simulink model "DriveSystemControl"  (R2023b)
settings: Solver=FixedStepAuto  StartTime=0.0  StopTime=Inf  FixedStep=0.001  RelTol=1e-3
PostLoadFcn:
  | if any(exist('dsrtsu_mdlpostloadfcn', 'file') ~= 0), dsrtsu_mdlpostloadfcn('Execute', bdroot); end
InitFcn:
  | , if any(exist('rtifpga_mdlclblib', 'file') ~= 0), rtifpga_mdlclblib('Init', bdroot); end,
  | , if any(exist('dsmpb_private', 'file') ~= 0), dsmpb_private('dsmpb_mdlclblib', 'Init', bdroot); end,
libraries: dsmpblib x2
(part 6 of 11)

== system DriveSystemControl/Bus Configuration (1) - Out/Simulated ECUs/Virya Controller CAN File 08082024/Telematics/RX/PDUs/TCU03/sigCurrentSensorFault ==
  sigCurrentSensorFault : Inport
  ISignal Value : Subsystem
  _sigCurrentSensorFault_ : BusSelector  OutputSignals=ISignal Value
  wires:
  sigCurrentSensorFault/1 -> _sigCurrentSensorFault_/1  "sigCurrentSensorFault"
  _sigCurrentSensorFault_/1 -> ISignal Value/1(ISignal Value)  "<ISignal Value>"

== system DriveSystemControl/Bus Configuration (1) - Out/Simulated ECUs/Virya Controller CAN File 08082024/Telematics/RX/PDUs/TCU03/sigEEPROMFailure ==
  sigEEPROMFailure : Inport
  ISignal Value : Subsystem
  _sigEEPROMFailure_ : BusSelector  OutputSignals=ISignal Value
  wires:
  sigEEPROMFailure/1 -> _sigEEPROMFailure_/1  "sigEEPROMFailure"
  _sigEEPROMFailure_/1 -> ISignal Value/1(ISignal Value)  "<ISignal Value>"

== system DriveSystemControl/Bus Configuration (1) - Out/Simulated ECUs/Virya Controller CAN File 08082024/Telematics/RX/PDUs/TCU03/sigHighPedalDisable ==
  sigHighPedalDisable : Inport
  ISignal Value : Subsystem
  _sigHighPedalDisable_ : BusSelector  OutputSignals=ISignal Value
  wires:
  sigHighPedalDisable/1 -> _sigHighPedalDisable_/1  "sigHighPedalDisable"
  _sigHighPedalDisable_/1 -> ISignal Value/1(ISignal Value)  "<ISignal Value>"

== system DriveSystemControl/Bus Configuration (1) - Out/Simulated ECUs/Virya Controller CAN File 08082024/Telematics/RX/PDUs/TCU03/sigInsulationResistanceLow ==
  sigInsulationResistanceLow : Inport
  ISignal Value : Subsystem
  _sigInsulationResistanceLow_ : BusSelector  OutputSignals=ISignal Value
  wires:
  sigInsulationResistanceLow/1 -> _sigInsulationResistanceLow_/1  "sigInsulationResistanceLow"
  _sigInsulationResistanceLow_/1 -> ISignal Value/1(ISignal Value)  "<ISignal Value>"

== system DriveSystemControl/Bus Configuration (1) - Out/Simulated ECUs/Virya Controller CAN File 08082024/Telematics/RX/PDUs/TCU03/sigMainContactorWelded ==
  sigMainContactorWelded : Inport
  ISignal Value : Subsystem
  _sigMainContactorWelded_ : BusSelector  OutputSignals=ISignal Value
  wires:
  sigMainContactorWelded/1 -> _sigMainContactorWelded_/1  "sigMainContactorWelded"
  _sigMainContactorWelded_/1 -> ISignal Value/1(ISignal Value)  "<ISignal Value>"

== system DriveSystemControl/Bus Configuration (1) - Out/Simulated ECUs/Virya Controller CAN File 08082024/Telematics/RX/PDUs/TCU03/sigMainContactordidnotClose ==
  sigMainContactordidnotClose : Inport
  ISignal Value : Subsystem
  _sigMainContactordidnotClose_ : BusSelector  OutputSignals=ISignal Value
  wires:
  sigMainContactordidnotClose/1 -> _sigMainContactordidnotClose_/1  "sigMainContactordidnotClose"
  _sigMainContactordidnotClose_/1 -> ISignal Value/1(ISignal Value)  "<ISignal Value>"

== system DriveSystemControl/Bus Configuration (1) - Out/Simulated ECUs/Virya Controller CAN File 08082024/Telematics/RX/PDUs/TCU03/sigMainOpenShort ==
  sigMainOpenShort : Inport
  ISignal Value : Subsystem
  _sigMainOpenShort_ : BusSelector  OutputSignals=ISignal Value
  wires:
  sigMainOpenShort/1 -> _sigMainOpenShort_/1  "sigMainOpenShort"
  _sigMainOpenShort_/1 -> ISignal Value/1(ISignal Value)  "<ISignal Value>"

== system DriveSystemControl/Bus Configuration (1) - Out/Simulated ECUs/Virya Controller CAN File 08082024/Telematics/RX/PDUs/TCU03/sigMotorCharacterization ==
  sigMotorCharacterization : Inport
  ISignal Value : Subsystem
  _sigMotorCharacterization_ : BusSelector  OutputSignals=ISignal Value
  wires:
  sigMotorCharacterization/1 -> _sigMotorCharacterization_/1  "sigMotorCharacterization"
  _sigMotorCharacterization_/1 -> ISignal Value/1(ISignal Value)  "<ISignal Value>"

== system DriveSystemControl/Bus Configuration (1) - Out/Simulated ECUs/Virya Controller CAN File 08082024/Telematics/RX/PDUs/TCU03/sigMotorPhaseOpen ==
  sigMotorPhaseOpen : Inport
  ISignal Value : Subsystem
  _sigMotorPhaseOpen_ : BusSelector  OutputSignals=ISignal Value
  wires:
  sigMotorPhaseOpen/1 -> _sigMotorPhaseOpen_/1  "sigMotorPhaseOpen"
  _sigMotorPhaseOpen_/1 -> ISignal Value/1(ISignal Value)  "<ISignal Value>"

== system DriveSystemControl/Bus Configuration (1) - Out/Simulated ECUs/Virya Controller CAN File 08082024/Telematics/RX/PDUs/TCU03/sigMotorTempHotCutback ==
  sigMotorTempHotCutback : Inport
  ISignal Value : Subsystem
  _sigMotorTempHotCutback_ : BusSelector  OutputSignals=ISignal Value
  wires:
  sigMotorTempHotCutback/1 -> _sigMotorTempHotCutback_/1  "sigMotorTempHotCutback"
  _sigMotorTempHotCutback_/1 -> ISignal Value/1(ISignal Value)  "<ISignal Value>"

== system DriveSystemControl/Bus Configuration (1) - Out/Simulated ECUs/Virya Controller CAN File 08082024/Telematics/RX/PDUs/TCU03/sigMotorTempSensorFault ==
  sigMotorTempSensorFault : Inport
  ISignal Value : Subsystem
  _sigMotorTempSensorFault_ : BusSelector  OutputSignals=ISignal Value
  wires:
  sigMotorTempSensorFault/1 -> _sigMotorTempSensorFault_/1  "sigMotorTempSensorFault"
  _sigMotorTempSensorFault_/1 -> ISignal Value/1(ISignal Value)  "<ISignal Value>"

== system DriveSystemControl/Bus Configuration (1) - Out/Simulated ECUs/Virya Controller CAN File 08082024/Telematics/RX/PDUs/TCU03/sigOEM_BatterySTOPSignal ==
  sigOEM_BatterySTOPSignal : Inport
  ISignal Value : Subsystem
  _sigOEM_BatterySTOPSignal_ : BusSelector  OutputSignals=ISignal Value
  wires:
  sigOEM_BatterySTOPSignal/1 -> _sigOEM_BatterySTOPSignal_/1  "sigOEM_BatterySTOPSignal"
  _sigOEM_BatterySTOPSignal_/1 -> ISignal Value/1(ISignal Value)  "<ISignal Value>"

== system DriveSystemControl/Bus Configuration (1) - Out/Simulated ECUs/Virya Controller CAN File 08082024/Telematics/RX/PDUs/TCU03/sigOEM_NoBatteryCAN ==
  sigOEM_NoBatteryCAN : Inport
  ISignal Value : Subsystem
  _sigOEM_NoBatteryCAN_ : BusSelector  OutputSignals=ISignal Value
  wires:
  sigOEM_NoBatteryCAN/1 -> _sigOEM_NoBatteryCAN_/1  "sigOEM_NoBatteryCAN"
  _sigOEM_NoBatteryCAN_/1 -> ISignal Value/1(ISignal Value)  "<ISignal Value>"

== system DriveSystemControl/Bus Configuration (1) - Out/Simulated ECUs/Virya Controller CAN File 08082024/Telematics/RX/PDUs/TCU03/sigOSGeneral ==
  sigOSGeneral : Inport
  ISignal Value : Subsystem
  _sigOSGeneral_ : BusSelector  OutputSignals=ISignal Value
  wires:
  sigOSGeneral/1 -> _sigOSGeneral_/1  "sigOSGeneral"
  _sigOSGeneral_/1 -> ISignal Value/1(ISignal Value)  "<ISignal Value>"

== system DriveSystemControl/Bus Configuration (1) - Out/Simulated ECUs/Virya Controller CAN File 08082024/Telematics/RX/PDUs/TCU03/sigPMACCommissioningNeeded ==
  sigPMACCommissioningNeeded : Inport
  ISignal Value : Subsystem
  _sigPMACCommissioningNeeded_ : BusSelector  OutputSignals=ISignal Value
  wires:
  sigPMACCommissioningNeeded/1 -> _sigPMACCommissioningNeeded_/1  "sigPMACCommissioningNeeded"
  _sigPMACCommissioningNeeded_/1 -> ISignal Value/1(ISignal Value)  "<ISignal Value>"

== system DriveSystemControl/Bus Configuration (1) - Out/Simulated ECUs/Virya Controller CAN File 08082024/Telematics/RX/PDUs/TCU03/sigParameterChangeFault ==
  sigParameterChangeFault : Inport
  ISignal Value : Subsystem
  _sigParameterChangeFault_ : BusSelector  OutputSignals=ISignal Value
  wires:
  sigParameterChangeFault/1 -> _sigParameterChangeFault_/1  "sigParameterChangeFault"
  _sigParameterChangeFault_/1 -> ISignal Value/1(ISignal Value)  "<ISignal Value>"

== system DriveSystemControl/Bus Configuration (1) - Out/Simulated ECUs/Virya Controller CAN File 08082024/Telematics/RX/PDUs/TCU03/sigPhasePWMMismatch ==
  sigPhasePWMMismatch : Inport
  ISignal Value : Subsystem
  _sigPhasePWMMismatch_ : BusSelector  OutputSignals=ISignal Value
  wires:
  sigPhasePWMMismatch/1 -> _sigPhasePWMMismatch_/1  "sigPhasePWMMismatch"
  _sigPhasePWMMismatch_/1 -> ISignal Value/1(ISignal Value)  "<ISignal Value>"

== system DriveSystemControl/Bus Configuration (1) - Out/Simulated ECUs/Virya Controller CAN File 08082024/Telematics/RX/PDUs/TCU03/sigPrechargeFailed ==
  sigPrechargeFailed : Inport
  ISignal Value : Subsystem
  _sigPrechargeFailed_ : BusSelector  OutputSignals=ISignal Value
  wires:
  sigPrechargeFailed/1 -> _sigPrechargeFailed_/1  "sigPrechargeFailed"
  _sigPrechargeFailed_/1 -> ISignal Value/1(ISignal Value)  "<ISignal Value>"

== system DriveSystemControl/Bus Configuration (1) - Out/Simulated ECUs/Virya Controller CAN File 08082024/Telematics/RX/PDUs/TCU03/sigSevereBPosOvervoltage ==
  sigSevereBPosOvervoltage : Inport
  ISignal Value : Subsystem
  _sigSevereBPosOvervoltage_ : BusSelector  OutputSignals=ISignal Value
  wires:
  sigSevereBPosOvervoltage/1 -> _sigSevereBPosOvervoltage_/1  "sigSevereBPosOvervoltage"
  _sigSevereBPosOvervoltage_/1 -> ISignal Value/1(ISignal Value)  "<ISignal Value>"

== system DriveSystemControl/Bus Configuration (1) - Out/Simulated ECUs/Virya Controller CAN File 08082024/Telematics/RX/PDUs/TCU03/sigSevereBPosUndervoltage ==
  sigSevereBPosUndervoltage : Inport
  ISignal Value : Subsystem
  _sigSevereBPosUndervoltage_ : BusSelector  OutputSignals=ISignal Value
  wires:
  sigSevereBPosUndervoltage/1 -> _sigSevereBPosUndervoltage_/1  "sigSevereBPosUndervoltage"
  _sigSevereBPosUndervoltage_/1 -> ISignal Value/1(ISignal Value)  "<ISignal Value>"

== system DriveSystemControl/Bus Configuration (1) - Out/Simulated ECUs/Virya Controller CAN File 08082024/Telematics/RX/PDUs/TCU03/sigSevereKSIOvervoltage ==
  sigSevereKSIOvervoltage : Inport
  ISignal Value : Subsystem
  _sigSevereKSIOvervoltage_ : BusSelector  OutputSignals=ISignal Value
  wires:
  sigSevereKSIOvervoltage/1 -> _sigSevereKSIOvervoltage_/1  "sigSevereKSIOvervoltage"
  _sigSevereKSIOvervoltage_/1 -> ISignal Value/1(ISignal Value)  "<ISignal Value>"

== system DriveSystemControl/Bus Configuration (1) - Out/Simulated ECUs/Virya Controller CAN File 08082024/Telematics/RX/PDUs/TCU03/sigSevereKSIUndervoltage ==
  sigSevereKSIUndervoltage : Inport
  ISignal Value : Subsystem
  _sigSevereKSIUndervoltage_ : BusSelector  OutputSignals=ISignal Value
  wires:
  sigSevereKSIUndervoltage/1 -> _sigSevereKSIUndervoltage_/1  "sigSevereKSIUndervoltage"
  _sigSevereKSIUndervoltage_/1 -> ISignal Value/1(ISignal Value)  "<ISignal Value>"

== system DriveSystemControl/Bus Configuration (1) - Out/Simulated ECUs/Virya Controller CAN File 08082024/Telematics/RX/PDUs/TCU03/sigSinCosMisalignment ==
  sigSinCosMisalignment : Inport
  ISignal Value : Subsystem
  _sigSinCosMisalignment_ : BusSelector  OutputSignals=ISignal Value
  wires:
  sigSinCosMisalignment/1 -> _sigSinCosMisalignment_/1  "sigSinCosMisalignment"
  _sigSinCosMisalignment_/1 -> ISignal Value/1(ISignal Value)  "<ISignal Value>"

== system DriveSystemControl/Bus Configuration (1) - Out/Simulated ECUs/Virya Controller CAN File 08082024/Telematics/RX/PDUs/TCU03/sigSinCosSensorFault ==
  sigSinCosSensorFault : Inport
  ISignal Value : Subsystem
  _sigSinCosSensorFault_ : BusSelector  OutputSignals=ISignal Value
  wires:
  sigSinCosSensorFault/1 -> _sigSinCosSensorFault_/1  "sigSinCosSensorFault"
  _sigSinCosSensorFault_/1 -> ISignal Value/1(ISignal Value)  "<ISignal Value>"

== system DriveSystemControl/Bus Configuration (1) - Out/Simulated ECUs/Virya Controller CAN File 08082024/Telematics/RX/PDUs/TCU03/sigStallDetected ==
  sigStallDetected : Inport
  ISignal Value : Subsystem
  _sigStallDetected_ : BusSelector  OutputSignals=ISignal Value
  wires:
  sigStallDetected/1 -> _sigStallDetected_/1  "sigStallDetected"
  _sigStallDetected_/1 -> ISignal Value/1(ISignal Value)  "<ISignal Value>"

== system DriveSystemControl/Bus Configuration (1) - Out/Simulated ECUs/Virya Controller CAN File 08082024/Telematics/RX/PDUs/TCU03/sigSupervisorFault ==
  sigSupervisorFault : Inport
  ISignal Value : Subsystem
  _sigSupervisorFault_ : BusSelector  OutputSignals=ISignal Value
  wires:
  sigSupervisorFault/1 -> _sigSupervisorFault_/1  "sigSupervisorFault"
  _sigSupervisorFault_/1 -> ISignal Value/1(ISignal Value)  "<ISignal Value>"

== system DriveSystemControl/Bus Configuration (1) - Out/Simulated ECUs/Virya Controller CAN File 08082024/Telematics/RX/PDUs/TCU03/sigThrottlewiperHigh ==
  sigThrottlewiperHigh : Inport
  ISignal Value : Subsystem
  _sigThrottlewiperHigh_ : BusSelector  OutputSignals=ISignal Value
  wires:
  sigThrottlewiperHigh/1 -> _sigThrottlewiperHigh_/1  "sigThrottlewiperHigh"
  _sigThrottlewiperHigh_/1 -> ISignal Value/1(ISignal Value)  "<ISignal Value>"

== system DriveSystemControl/Bus Configuration (1) - Out/Simulated ECUs/Virya Controller CAN File 08082024/Telematics/RX/PDUs/TCU03/sigThrottlewiperLow ==
  sigThrottlewiperLow : Inport
  ISignal Value : Subsystem
  _sigThrottlewiperLow_ : BusSelector  OutputSignals=ISignal Value
  wires:
  sigThrottlewiperLow/1 -> _sigThrottlewiperLow_/1  "sigThrottlewiperLow"
  _sigThrottlewiperLow_/1 -> ISignal Value/1(ISignal Value)  "<ISignal Value>"

== system DriveSystemControl/Bus Configuration (1) - Out/Simulated ECUs/Virya Controller CAN File 08082024/Telematics/RX/PDUs/TCU03/sigVCLRunTimeError ==
  sigVCLRunTimeError : Inport
  ISignal Value : Subsystem
  _sigVCLRunTimeError_ : BusSelector  OutputSignals=ISignal Value
  wires:
  sigVCLRunTimeError/1 -> _sigVCLRunTimeError_/1  "sigVCLRunTimeError"
  _sigVCLRunTimeError_/1 -> ISignal Value/1(ISignal Value)  "<ISignal Value>"

== system DriveSystemControl/Bus Configuration (1) - Out/Simulated ECUs/Virya Controller CAN File 08082024/Telematics/RX/PDUs/TCU04/sigMCU5_DriveMode ==
  sigMCU5_DriveMode : Inport
  ISignal Value : Subsystem
  _sigMCU5_DriveMode_ : BusSelector  OutputSignals=ISignal Value
  wires:
  sigMCU5_DriveMode/1 -> _sigMCU5_DriveMode_/1  "sigMCU5_DriveMode"
  _sigMCU5_DriveMode_/1 -> ISignal Value/1(ISignal Value)  "<ISignal Value>"

== system DriveSystemControl/Bus Configuration (1) - Out/Simulated ECUs/Virya Controller CAN File 08082024/Telematics/RX/PDUs/TCU04/sigMCU5_Efficiency ==
  sigMCU5_Efficiency : Inport
  ISignal Value : Subsystem
  _sigMCU5_Efficiency_ : BusSelector  OutputSignals=ISignal Value
  wires:
  sigMCU5_Efficiency/1 -> _sigMCU5_Efficiency_/1  "sigMCU5_Efficiency"
  _sigMCU5_Efficiency_/1 -> ISignal Value/1(ISignal Value)  "<ISignal Value>"

== system DriveSystemControl/Bus Configuration (1) - Out/Simulated ECUs/Virya Controller CAN File 08082024/Telematics/RX/PDUs/TCU04/sigMCU5_Hillhold ==
  sigMCU5_Hillhold : Inport
  ISignal Value : Subsystem
  _sigMCU5_Hillhold_ : BusSelector  OutputSignals=ISignal Value
  wires:
  sigMCU5_Hillhold/1 -> _sigMCU5_Hillhold_/1  "sigMCU5_Hillhold"
  _sigMCU5_Hillhold_/1 -> ISignal Value/1(ISignal Value)  "<ISignal Value>"

== system DriveSystemControl/Bus Configuration (1) - Out/Simulated ECUs/Virya Controller CAN File 08082024/Telematics/RX/PDUs/TCU04/sigMCU5_RegenFlag ==
  sigMCU5_RegenFlag : Inport
  ISignal Value : Subsystem
  _sigMCU5_RegenFlag_ : BusSelector  OutputSignals=ISignal Value
  wires:
  sigMCU5_RegenFlag/1 -> _sigMCU5_RegenFlag_/1  "sigMCU5_RegenFlag"
  _sigMCU5_RegenFlag_/1 -> ISignal Value/1(ISignal Value)  "<ISignal Value>"

== system DriveSystemControl/Bus Configuration (1) - Out/Simulated ECUs/Virya Controller CAN File 08082024/Telematics/RX/PDUs/TCU04/sigMCU5_Speed ==
  sigMCU5_Speed : Inport
  ISignal Value : Subsystem
  _sigMCU5_Speed_ : BusSelector  OutputSignals=ISignal Value
  wires:
  sigMCU5_Speed/1 -> _sigMCU5_Speed_/1  "sigMCU5_Speed"
  _sigMCU5_Speed_/1 -> ISignal Value/1(ISignal Value)  "<ISignal Value>"

== system DriveSystemControl/Bus Configuration (1) - Out/Simulated ECUs/Virya Controller CAN File 08082024/Telematics/RX/PDUs/TCU05/sigMCU6_Odometer ==
  sigMCU6_Odometer : Inport
  ISignal Value : Subsystem
  _sigMCU6_Odometer_ : BusSelector  OutputSignals=ISignal Value
  wires:
  sigMCU6_Odometer/1 -> _sigMCU6_Odometer_/1  "sigMCU6_Odometer"
  _sigMCU6_Odometer_/1 -> ISignal Value/1(ISignal Value)  "<ISignal Value>"

== system DriveSystemControl/Bus Configuration (1) - In/Manipulation/Virya Controller CAN File 08082024/WIP/CANChannel/PDUs/BMS01/sigBatteryMalfunctionLight/Feature Switch ==
  Const_sigBatteryMalfunctionLight Countdown Start Value : Constant  Value=0  OutDataTypeStr=uint32
  Const_sigBatteryMalfunctionLight Feature Switch : Constant  Value=0  OutDataTypeStr=uint32
  _Feature Switch_ : BusCreator  Inputs=2
  Feature Switch : Outport
  wires:
  _Feature Switch_/1 -> Feature Switch/1  "Feature Switch"
  Const_sigBatteryMalfunctionLight Countdown Start Value/1 -> _Feature Switch_/1  "sigBatteryMalfunctionLight Countdown Start Value"
  Const_sigBatteryMalfunctionLight Feature Switch/1 -> _Feature Switch_/2  "sigBatteryMalfunctionLight Feature Switch"

== system DriveSystemControl/Bus Configuration (1) - In/Manipulation/Virya Controller CAN File 08082024/WIP/CANChannel/PDUs/BMS01/sigBatteryMalfunctionLight/ISignal Overwrite Value ==
  Const_sigBatteryMalfunctionLight Overwrite Value : Constant  Value=0  OutDataTypeStr=uint8
  _ISignal Overwrite Value_ : BusCreator  Inputs=1
  ISignal Overwrite Value : Outport
  wires:
  _ISignal Overwrite Value_/1 -> ISignal Overwrite Value/1  "ISignal Overwrite Value"
  Const_sigBatteryMalfunctionLight Overwrite Value/1 -> _ISignal Overwrite Value_/1  "sigBatteryMalfunctionLight Overwrite Value"

== system DriveSystemControl/Bus Configuration (1) - In/Manipulation/Virya Controller CAN File 08082024/WIP/CANChannel/PDUs/BMS01/sigKeyOnIndicator/Feature Switch ==
  Const_sigKeyOnIndicator Countdown Start Value : Constant  Value=0  OutDataTypeStr=uint32
  Const_sigKeyOnIndicator Feature Switch : Constant  Value=0  OutDataTypeStr=uint32
  _Feature Switch_ : BusCreator  Inputs=2
  Feature Switch : Outport
  wires:
  _Feature Switch_/1 -> Feature Switch/1  "Feature Switch"
  Const_sigKeyOnIndicator Countdown Start Value/1 -> _Feature Switch_/1  "sigKeyOnIndicator Countdown Start Value"
  Const_sigKeyOnIndicator Feature Switch/1 -> _Feature Switch_/2  "sigKeyOnIndicator Feature Switch"

== system DriveSystemControl/Bus Configuration (1) - In/Manipulation/Virya Controller CAN File 08082024/WIP/CANChannel/PDUs/BMS01/sigKeyOnIndicator/ISignal Overwrite Value ==
  Const_sigKeyOnIndicator Overwrite Value : Constant  Value=0  OutDataTypeStr=uint8
  _ISignal Overwrite Value_ : BusCreator  Inputs=1
  ISignal Overwrite Value : Outport
  wires:
  _ISignal Overwrite Value_/1 -> ISignal Overwrite Value/1  "ISignal Overwrite Value"
  Const_sigKeyOnIndicator Overwrite Value/1 -> _ISignal Overwrite Value_/1  "sigKeyOnIndicator Overwrite Value"

== system DriveSystemControl/Bus Configuration (1) - In/Manipulation/Virya Controller CAN File 08082024/WIP/CANChannel/PDUs/BMS01/sigStateOfCharge/Feature Switch ==
  Const_sigStateOfCharge Countdown Start Value : Constant  Value=0  OutDataTypeStr=uint32
  Const_sigStateOfCharge Feature Switch : Constant  Value=0  OutDataTypeStr=uint32
  _Feature Switch_ : BusCreator  Inputs=2
  Feature Switch : Outport
  wires:
  _Feature Switch_/1 -> Feature Switch/1  "Feature Switch"
  Const_sigStateOfCharge Countdown Start Value/1 -> _Feature Switch_/1  "sigStateOfCharge Countdown Start Value"
  Const_sigStateOfCharge Feature Switch/1 -> _Feature Switch_/2  "sigStateOfCharge Feature Switch"

== system DriveSystemControl/Bus Configuration (1) - In/Manipulation/Virya Controller CAN File 08082024/WIP/CANChannel/PDUs/BMS01/sigStateOfCharge/ISignal Overwrite Value ==
  Const_sigStateOfCharge Overwrite Value : Constant  Value=0  OutDataTypeStr=uint8
  _ISignal Overwrite Value_ : BusCreator  Inputs=1
  ISignal Overwrite Value : Outport
  wires:
  _ISignal Overwrite Value_/1 -> ISignal Overwrite Value/1  "ISignal Overwrite Value"
  Const_sigStateOfCharge Overwrite Value/1 -> _ISignal Overwrite Value_/1  "sigStateOfCharge Overwrite Value"

== system DriveSystemControl/Bus Configuration (1) - In/Manipulation/Virya Controller CAN File 08082024/WIP/CANChannel/PDUs/BMS02/sigBatteryCurrent/Feature Switch ==
  Const_sigBatteryCurrent Countdown Start Value : Constant  Value=0  OutDataTypeStr=uint32
  Const_sigBatteryCurrent Feature Switch : Constant  Value=0  OutDataTypeStr=uint32
  _Feature Switch_ : BusCreator  Inputs=2
  Feature Switch : Outport
  wires:
  _Feature Switch_/1 -> Feature Switch/1  "Feature Switch"
  Const_sigBatteryCurrent Countdown Start Value/1 -> _Feature Switch_/1  "sigBatteryCurrent Countdown Start Value"
  Const_sigBatteryCurrent Feature Switch/1 -> _Feature Switch_/2  "sigBatteryCurrent Feature Switch"

== system DriveSystemControl/Bus Configuration (1) - In/Manipulation/Virya Controller CAN File 08082024/WIP/CANChannel/PDUs/BMS02/sigBatteryCurrent/ISignal Overwrite Value ==
  Const_sigBatteryCurrent Overwrite Value : Constant  Value=0  OutDataTypeStr=double
  _ISignal Overwrite Value_ : BusCreator  Inputs=1
  ISignal Overwrite Value : Outport
  wires:
  _ISignal Overwrite Value_/1 -> ISignal Overwrite Value/1  "ISignal Overwrite Value"
  Const_sigBatteryCurrent Overwrite Value/1 -> _ISignal Overwrite Value_/1  "sigBatteryCurrent Overwrite Value"

== system DriveSystemControl/Bus Configuration (1) - In/Manipulation/Virya Controller CAN File 08082024/WIP/CANChannel/PDUs/BMS02/sigDriveCurrentLimit/Feature Switch ==
  Const_sigDriveCurrentLimit Countdown Start Value : Constant  Value=0  OutDataTypeStr=uint32
  Const_sigDriveCurrentLimit Feature Switch : Constant  Value=0  OutDataTypeStr=uint32
  _Feature Switch_ : BusCreator  Inputs=2
  Feature Switch : Outport
  wires:
  _Feature Switch_/1 -> Feature Switch/1  "Feature Switch"
  Const_sigDriveCurrentLimit Countdown Start Value/1 -> _Feature Switch_/1  "sigDriveCurrentLimit Countdown Start Value"
  Const_sigDriveCurrentLimit Feature Switch/1 -> _Feature Switch_/2  "sigDriveCurrentLimit Feature Switch"

== system DriveSystemControl/Bus Configuration (1) - In/Manipulation/Virya Controller CAN File 08082024/WIP/CANChannel/PDUs/BMS02/sigDriveCurrentLimit/ISignal Overwrite Value ==
  Const_sigDriveCurrentLimit Overwrite Value : Constant  Value=0  OutDataTypeStr=uint8
  _ISignal Overwrite Value_ : BusCreator  Inputs=1
  ISignal Overwrite Value : Outport
  wires:
  _ISignal Overwrite Value_/1 -> ISignal Overwrite Value/1  "ISignal Overwrite Value"
  Const_sigDriveCurrentLimit Overwrite Value/1 -> _ISignal Overwrite Value_/1  "sigDriveCurrentLimit Overwrite Value"

== system DriveSystemControl/Bus Configuration (1) - In/Manipulation/Virya Controller CAN File 08082024/WIP/CANChannel/PDUs/BMS02/sigRegenCurrentLimit/Feature Switch ==
  Const_sigRegenCurrentLimit Countdown Start Value : Constant  Value=0  OutDataTypeStr=uint32
  Const_sigRegenCurrentLimit Feature Switch : Constant  Value=0  OutDataTypeStr=uint32
  _Feature Switch_ : BusCreator  Inputs=2
  Feature Switch : Outport
  wires:
  _Feature Switch_/1 -> Feature Switch/1  "Feature Switch"
  Const_sigRegenCurrentLimit Countdown Start Value/1 -> _Feature Switch_/1  "sigRegenCurrentLimit Countdown Start Value"
  Const_sigRegenCurrentLimit Feature Switch/1 -> _Feature Switch_/2  "sigRegenCurrentLimit Feature Switch"

== system DriveSystemControl/Bus Configuration (1) - In/Manipulation/Virya Controller CAN File 08082024/WIP/CANChannel/PDUs/BMS02/sigRegenCurrentLimit/ISignal Overwrite Value ==
  Const_sigRegenCurrentLimit Overwrite Value : Constant  Value=0  OutDataTypeStr=uint8
  _ISignal Overwrite Value_ : BusCreator  Inputs=1
  ISignal Overwrite Value : Outport
  wires:
  _ISignal Overwrite Value_/1 -> ISignal Overwrite Value/1  "ISignal Overwrite Value"
  Const_sigRegenCurrentLimit Overwrite Value/1 -> _ISignal Overwrite Value_/1  "sigRegenCurrentLimit Overwrite Value"

== system DriveSystemControl/Bus Configuration (1) - In/Manipulation/Virya Controller CAN File 08082024/WIP/CANChannel/PDUs/BMS02/sigVehicleModeRequest/Feature Switch ==
  Const_sigVehicleModeRequest Countdown Start Value : Constant  Value=0  OutDataTypeStr=uint32
  Const_sigVehicleModeRequest Feature Switch : Constant  Value=0  OutDataTypeStr=uint32
  _Feature Switch_ : BusCreator  Inputs=2
  Feature Switch : Outport
  wires:
  _Feature Switch_/1 -> Feature Switch/1  "Feature Switch"
  Const_sigVehicleModeRequest Countdown Start Value/1 -> _Feature Switch_/1  "sigVehicleModeRequest Countdown Start Value"
  Const_sigVehicleModeRequest Feature Switch/1 -> _Feature Switch_/2  "sigVehicleModeRequest Feature Switch"

== system DriveSystemControl/Bus Configuration (1) - In/Manipulation/Virya Controller CAN File 08082024/WIP/CANChannel/PDUs/BMS02/sigVehicleModeRequest/ISignal Overwrite Value ==
  Const_sigVehicleModeRequest Overwrite Value : Constant  Value=0  OutDataTypeStr=uint8
  _ISignal Overwrite Value_ : BusCreator  Inputs=1
  ISignal Overwrite Value : Outport
  wires:
  _ISignal Overwrite Value_/1 -> ISignal Overwrite Value/1  "ISignal Overwrite Value"
  Const_sigVehicleModeRequest Overwrite Value/1 -> _ISignal Overwrite Value_/1  "sigVehicleModeRequest Overwrite Value"

== system DriveSystemControl/Bus Configuration (1) - In/Manipulation/Virya Controller CAN File 08082024/WIP/CANChannel/PDUs/MainController/CCU_heartBeat/Feature Switch ==
  Const_CCU_heartBeat Countdown Start Value : Constant  Value=0  OutDataTypeStr=uint32
  Const_CCU_heartBeat Feature Switch : Constant  Value=0  OutDataTypeStr=uint32
  _Feature Switch_ : BusCreator  Inputs=2
  Feature Switch : Outport
  wires:
  _Feature Switch_/1 -> Feature Switch/1  "Feature Switch"
  Const_CCU_heartBeat Countdown Start Value/1 -> _Feature Switch_/1  "CCU_heartBeat Countdown Start Value"
  Const_CCU_heartBeat Feature Switch/1 -> _Feature Switch_/2  "CCU_heartBeat Feature Switch"

== system DriveSystemControl/Bus Configuration (1) - In/Manipulation/Virya Controller CAN File 08082024/WIP/CANChannel/PDUs/MainController/CCU_heartBeat/ISignal Overwrite Value ==
  Const_CCU_heartBeat Overwrite Value : Constant  Value=0  OutDataTypeStr=uint8
  _ISignal Overwrite Value_ : BusCreator  Inputs=1
  ISignal Overwrite Value : Outport
  wires:
  _ISignal Overwrite Value_/1 -> ISignal Overwrite Value/1  "ISignal Overwrite Value"
  Const_CCU_heartBeat Overwrite Value/1 -> _ISignal Overwrite Value_/1  "CCU_heartBeat Overwrite Value"

== system DriveSystemControl/Bus Configuration (1) - In/Manipulation/Virya Controller CAN File 08082024/WIP/CANChannel/PDUs/MainController/notUsed/Feature Switch ==
  Const_notUsed Countdown Start Value : Constant  Value=0  OutDataTypeStr=uint32
  Const_notUsed Feature Switch : Constant  Value=0  OutDataTypeStr=uint32
  _Feature Switch_ : BusCreator  Inputs=2
  Feature Switch : Outport
  wires:
  _Feature Switch_/1 -> Feature Switch/1  "Feature Switch"
  Const_notUsed Countdown Start Value/1 -> _Feature Switch_/1  "notUsed Countdown Start Value"
  Const_notUsed Feature Switch/1 -> _Feature Switch_/2  "notUsed Feature Switch"

== system DriveSystemControl/Bus Configuration (1) - In/Manipulation/Virya Controller CAN File 08082024/WIP/CANChannel/PDUs/MainController/notUsed/ISignal Overwrite Value ==
  Const_notUsed Overwrite Value : Constant  Value=0  OutDataTypeStr=uint8
  _ISignal Overwrite Value_ : BusCreator  Inputs=1
  ISignal Overwrite Value : Outport
  wires:
  _ISignal Overwrite Value_/1 -> ISignal Overwrite Value/1  "ISignal Overwrite Value"
  Const_notUsed Overwrite Value/1 -> _ISignal Overwrite Value_/1  "notUsed Overwrite Value"

== system DriveSystemControl/Bus Configuration (1) - In/Manipulation/Virya Controller CAN File 08082024/WIP/CANChannel/PDUs/MainController/setAutoParkBreak/Feature Switch ==
  Const_setAutoParkBreak Countdown Start Value : Constant  Value=0  OutDataTypeStr=uint32
  Const_setAutoParkBreak Feature Switch : Constant  Value=0  OutDataTypeStr=uint32
  _Feature Switch_ : BusCreator  Inputs=2
  Feature Switch : Outport
  wires:
  _Feature Switch_/1 -> Feature Switch/1  "Feature Switch"
  Const_setAutoParkBreak Countdown Start Value/1 -> _Feature Switch_/1  "setAutoParkBreak Countdown Start Value"
  Const_setAutoParkBreak Feature Switch/1 -> _Feature Switch_/2  "setAutoParkBreak Feature Switch"

== system DriveSystemControl/Bus Configuration (1) - In/Manipulation/Virya Controller CAN File 08082024/WIP/CANChannel/PDUs/MainController/setAutoParkBreak/ISignal Overwrite Value ==
  Const_setAutoParkBreak Overwrite Value : Constant  Value=0  OutDataTypeStr=uint8
  _ISignal Overwrite Value_ : BusCreator  Inputs=1
  ISignal Overwrite Value : Outport
  wires:
  _ISignal Overwrite Value_/1 -> ISignal Overwrite Value/1  "ISignal Overwrite Value"
  Const_setAutoParkBreak Overwrite Value/1 -> _ISignal Overwrite Value_/1  "setAutoParkBreak Overwrite Value"

== system DriveSystemControl/Bus Configuration (1) - In/Manipulation/Virya Controller CAN File 08082024/WIP/CANChannel/PDUs/MainController/setBreake/Feature Switch ==
  Const_setBreake Countdown Start Value : Constant  Value=0  OutDataTypeStr=uint32
  Const_setBreake Feature Switch : Constant  Value=0  OutDataTypeStr=uint32
  _Feature Switch_ : BusCreator  Inputs=2
  Feature Switch : Outport
  wires:
  _Feature Switch_/1 -> Feature Switch/1  "Feature Switch"
  Const_setBreake Countdown Start Value/1 -> _Feature Switch_/1  "setBreake Countdown Start Value"
  Const_setBreake Feature Switch/1 -> _Feature Switch_/2  "setBreake Feature Switch"

== system DriveSystemControl/Bus Configuration (1) - In/Manipulation/Virya Controller CAN File 08082024/WIP/CANChannel/PDUs/MainController/setBreake/ISignal Overwrite Value ==
  Const_setBreake Overwrite Value : Constant  Value=0  OutDataTypeStr=uint8
  _ISignal Overwrite Value_ : BusCreator  Inputs=1
  ISignal Overwrite Value : Outport
  wires:
  _ISignal Overwrite Value_/1 -> ISignal Overwrite Value/1  "ISignal Overwrite Value"
  Const_setBreake Overwrite Value/1 -> _ISignal Overwrite Value_/1  "setBreake Overwrite Value"

== system DriveSystemControl/Bus Configuration (1) - In/Manipulation/Virya Controller CAN File 08082024/WIP/CANChannel/PDUs/MainController/setDirection/Feature Switch ==
  Const_setDirection Countdown Start Value : Constant  Value=0  OutDataTypeStr=uint32
  Const_setDirection Feature Switch : Constant  Value=0  OutDataTypeStr=uint32
  _Feature Switch_ : BusCreator  Inputs=2
  Feature Switch : Outport
  wires:
  _Feature Switch_/1 -> Feature Switch/1  "Feature Switch"
  Const_setDirection Countdown Start Value/1 -> _Feature Switch_/1  "setDirection Countdown Start Value"
  Const_setDirection Feature Switch/1 -> _Feature Switch_/2  "setDirection Feature Switch"

== system DriveSystemControl/Bus Configuration (1) - In/Manipulation/Virya Controller CAN File 08082024/WIP/CANChannel/PDUs/MainController/setDirection/ISignal Overwrite Value ==
  Const_setDirection Overwrite Value : Constant  Value=0  OutDataTypeStr=uint8
  _ISignal Overwrite Value_ : BusCreator  Inputs=1
  ISignal Overwrite Value : Outport
  wires:
  _ISignal Overwrite Value_/1 -> ISignal Overwrite Value/1  "ISignal Overwrite Value"
  Const_setDirection Overwrite Value/1 -> _ISignal Overwrite Value_/1  "setDirection Overwrite Value"

== system DriveSystemControl/Bus Configuration (1) - In/Manipulation/Virya Controller CAN File 08082024/WIP/CANChannel/PDUs/MainController/setDriveMode/Feature Switch ==
  Const_setDriveMode Countdown Start Value : Constant  Value=0  OutDataTypeStr=uint32
  Const_setDriveMode Feature Switch : Constant  Value=0  OutDataTypeStr=uint32
  _Feature Switch_ : BusCreator  Inputs=2
  Feature Switch : Outport
  wires:
  _Feature Switch_/1 -> Feature Switch/1  "Feature Switch"
  Const_setDriveMode Countdown Start Value/1 -> _Feature Switch_/1  "setDriveMode Countdown Start Value"
  Const_setDriveMode Feature Switch/1 -> _Feature Switch_/2  "setDriveMode Feature Switch"

== system DriveSystemControl/Bus Configuration (1) - In/Manipulation/Virya Controller CAN File 08082024/WIP/CANChannel/PDUs/MainController/setDriveMode/ISignal Overwrite Value ==
  Const_setDriveMode Overwrite Value : Constant  Value=0  OutDataTypeStr=uint8
  _ISignal Overwrite Value_ : BusCreator  Inputs=1
  ISignal Overwrite Value : Outport
  wires:
  _ISignal Overwrite Value_/1 -> ISignal Overwrite Value/1  "ISignal Overwrite Value"
  Const_setDriveMode Overwrite Value/1 -> _ISignal Overwrite Value_/1  "setDriveMode Overwrite Value"

== system DriveSystemControl/Bus Configuration (1) - In/Manipulation/Virya Controller CAN File 08082024/WIP/CANChannel/PDUs/MainController/setVelocity/Feature Switch ==
  Const_setVelocity Countdown Start Value : Constant  Value=0  OutDataTypeStr=uint32
  Const_setVelocity Feature Switch : Constant  Value=0  OutDataTypeStr=uint32
  _Feature Switch_ : BusCreator  Inputs=2
  Feature Switch : Outport
  wires:
  _Feature Switch_/1 -> Feature Switch/1  "Feature Switch"
  Const_setVelocity Countdown Start Value/1 -> _Feature Switch_/1  "setVelocity Countdown Start Value"
  Const_setVelocity Feature Switch/1 -> _Feature Switch_/2  "setVelocity Feature Switch"

== system DriveSystemControl/Bus Configuration (1) - In/Manipulation/Virya Controller CAN File 08082024/WIP/CANChannel/PDUs/MainController/setVelocity/ISignal Overwrite Value ==
  Const_setVelocity Overwrite Value : Constant  Value=0  OutDataTypeStr=uint8
  _ISignal Overwrite Value_ : BusCreator  Inputs=1
  ISignal Overwrite Value : Outport
  wires:
  _ISignal Overwrite Value_/1 -> ISignal Overwrite Value/1  "ISignal Overwrite Value"
  Const_setVelocity Overwrite Value/1 -> _ISignal Overwrite Value_/1  "setVelocity Overwrite Value"

== system DriveSystemControl/Bus Configuration (1) - In/Manipulation/Virya Controller CAN File 08082024/WIP/CANChannel/PDUs/MainController/steeringPower/Feature Switch ==
  Const_steeringPower Countdown Start Value : Constant  Value=0  OutDataTypeStr=uint32
  Const_steeringPower Feature Switch : Constant  Value=0  OutDataTypeStr=uint32
  _Feature Switch_ : BusCreator  Inputs=2
  Feature Switch : Outport
  wires:
  _Feature Switch_/1 -> Feature Switch/1  "Feature Switch"
  Const_steeringPower Countdown Start Value/1 -> _Feature Switch_/1  "steeringPower Countdown Start Value"
  Const_steeringPower Feature Switch/1 -> _Feature Switch_/2  "steeringPower Feature Switch"

== system DriveSystemControl/Bus Configuration (1) - In/Manipulation/Virya Controller CAN File 08082024/WIP/CANChannel/PDUs/MainController/steeringPower/ISignal Overwrite Value ==
  Const_steeringPower Overwrite Value : Constant  Value=0  OutDataTypeStr=uint8
  _ISignal Overwrite Value_ : BusCreator  Inputs=1
  ISignal Overwrite Value : Outport
  wires:
  _ISignal Overwrite Value_/1 -> ISignal Overwrite Value/1  "ISignal Overwrite Value"
  Const_steeringPower Overwrite Value/1 -> _ISignal Overwrite Value_/1  "steeringPower Overwrite Value"

== system DriveSystemControl/Bus Configuration (1) - In/Manipulation/Virya Controller CAN File 08082024/WIP/CANChannel/PDUs/TCU01/sigBrake/Feature Switch ==
  Const_sigBrake Countdown Start Value : Constant  Value=0  OutDataTypeStr=uint32
  Const_sigBrake Feature Switch : Constant  Value=0  OutDataTypeStr=uint32
  _Feature Switch_ : BusCreator  Inputs=2
  Feature Switch : Outport
  wires:
  _Feature Switch_/1 -> Feature Switch/1  "Feature Switch"
  Const_sigBrake Countdown Start Value/1 -> _Feature Switch_/1  "sigBrake Countdown Start Value"
  Const_sigBrake Feature Switch/1 -> _Feature Switch_/2  "sigBrake Feature Switch"

== system DriveSystemControl/Bus Configuration (1) - In/Manipulation/Virya Controller CAN File 08082024/WIP/CANChannel/PDUs/TCU01/sigBrake/ISignal Overwrite Value ==
  Const_sigBrake Overwrite Value : Constant  Value=0  OutDataTypeStr=uint8
  _ISignal Overwrite Value_ : BusCreator  Inputs=1
  ISignal Overwrite Value : Outport
  wires:
  _ISignal Overwrite Value_/1 -> ISignal Overwrite Value/1  "ISignal Overwrite Value"
  Const_sigBrake Overwrite Value/1 -> _ISignal Overwrite Value_/1  "sigBrake Overwrite Value"

== system DriveSystemControl/Bus Configuration (1) - In/Manipulation/Virya Controller CAN File 08082024/WIP/CANChannel/PDUs/TCU01/sigControllerTemperature/Feature Switch ==
  Const_sigControllerTemperature Countdown Start Value : Constant  Value=0  OutDataTypeStr=uint32
  Const_sigControllerTemperature Feature Switch : Constant  Value=0  OutDataTypeStr=uint32
  _Feature Switch_ : BusCreator  Inputs=2
  Feature Switch : Outport
  wires:
  _Feature Switch_/1 -> Feature Switch/1  "Feature Switch"
  Const_sigControllerTemperature Countdown Start Value/1 -> _Feature Switch_/1  "sigControllerTemperature Countdown Start Value"
  Const_sigControllerTemperature Feature Switch/1 -> _Feature Switch_/2  "sigControllerTemperature Feature Switch"

== system DriveSystemControl/Bus Configuration (1) - In/Manipulation/Virya Controller CAN File 08082024/WIP/CANChannel/PDUs/TCU01/sigControllerTemperature/ISignal Overwrite Value ==
  Const_sigControllerTemperature Overwrite Value : Constant  Value=0  OutDataTypeStr=int8
  _ISignal Overwrite Value_ : BusCreator  Inputs=1
  ISignal Overwrite Value : Outport
  wires:
  _ISignal Overwrite Value_/1 -> ISignal Overwrite Value/1  "ISignal Overwrite Value"
  Const_sigControllerTemperature Overwrite Value/1 -> _ISignal Overwrite Value_/1  "sigControllerTemperature Overwrite Value"

== system DriveSystemControl/Bus Configuration (1) - In/Manipulation/Virya Controller CAN File 08082024/WIP/CANChannel/PDUs/TCU01/sigDriveMode/Feature Switch ==
  Const_sigDriveMode Countdown Start Value : Constant  Value=0  OutDataTypeStr=uint32
  Const_sigDriveMode Feature Switch : Constant  Value=0  OutDataTypeStr=uint32
  _Feature Switch_ : BusCreator  Inputs=2
  Feature Switch : Outport
  wires:
  _Feature Switch_/1 -> Feature Switch/1  "Feature Switch"
  Const_sigDriveMode Countdown Start Value/1 -> _Feature Switch_/1  "sigDriveMode Countdown Start Value"
  Const_sigDriveMode Feature Switch/1 -> _Feature Switch_/2  "sigDriveMode Feature Switch"

== system DriveSystemControl/Bus Configuration (1) - In/Manipulation/Virya Controller CAN File 08082024/WIP/CANChannel/PDUs/TCU01/sigDriveMode/ISignal Overwrite Value ==
  Const_sigDriveMode Overwrite Value : Constant  Value=0  OutDataTypeStr=uint8
  _ISignal Overwrite Value_ : BusCreator  Inputs=1
  ISignal Overwrite Value : Outport
  wires:
  _ISignal Overwrite Value_/1 -> ISignal Overwrite Value/1  "ISignal Overwrite Value"
  Const_sigDriveMode Overwrite Value/1 -> _ISignal Overwrite Value_/1  "sigDriveMode Overwrite Value"

== system DriveSystemControl/Bus Configuration (1) - In/Manipulation/Virya Controller CAN File 08082024/WIP/CANChannel/PDUs/TCU01/sigMotorTemperature/Feature Switch ==
  Const_sigMotorTemperature Countdown Start Value : Constant  Value=0  OutDataTypeStr=uint32
  Const_sigMotorTemperature Feature Switch : Constant  Value=0  OutDataTypeStr=uint32
  _Feature Switch_ : BusCreator  Inputs=2
  Feature Switch : Outport
  wires:
  _Feature Switch_/1 -> Feature Switch/1  "Feature Switch"
  Const_sigMotorTemperature Countdown Start Value/1 -> _Feature Switch_/1  "sigMotorTemperature Countdown Start Value"
  Const_sigMotorTemperature Feature Switch/1 -> _Feature Switch_/2  "sigMotorTemperature Feature Switch"

== system DriveSystemControl/Bus Configuration (1) - In/Manipulation/Virya Controller CAN File 08082024/WIP/CANChannel/PDUs/TCU01/sigMotorTemperature/ISignal Overwrite Value ==
  Const_sigMotorTemperature Overwrite Value : Constant  Value=-50  OutDataTypeStr=int16
  _ISignal Overwrite Value_ : BusCreator  Inputs=1
  ISignal Overwrite Value : Outport
  wires:
  _ISignal Overwrite Value_/1 -> ISignal Overwrite Value/1  "ISignal Overwrite Value"
  Const_sigMotorTemperature Overwrite Value/1 -> _ISignal Overwrite Value_/1  "sigMotorTemperature Overwrite Value"

== system DriveSystemControl/Bus Configuration (1) - In/Manipulation/Virya Controller CAN File 08082024/WIP/CANChannel/PDUs/TCU01/sigRMSCurrent/Feature Switch ==
  Const_sigRMSCurrent Countdown Start Value : Constant  Value=0  OutDataTypeStr=uint32
  Const_sigRMSCurrent Feature Switch : Constant  Value=0  OutDataTypeStr=uint32
  _Feature Switch_ : BusCreator  Inputs=2
  Feature Switch : Outport
  wires:
  _Feature Switch_/1 -> Feature Switch/1  "Feature Switch"
  Const_sigRMSCurrent Countdown Start Value/1 -> _Feature Switch_/1  "sigRMSCurrent Countdown Start Value"
  Const_sigRMSCurrent Feature Switch/1 -> _Feature Switch_/2  "sigRMSCurrent Feature Switch"

== system DriveSystemControl/Bus Configuration (1) - In/Manipulation/Virya Controller CAN File 08082024/WIP/CANChannel/PDUs/TCU01/sigRMSCurrent/ISignal Overwrite Value ==
  Const_sigRMSCurrent Overwrite Value : Constant  Value=0  OutDataTypeStr=double
  _ISignal Overwrite Value_ : BusCreator  Inputs=1
  ISignal Overwrite Value : Outport
  wires:
  _ISignal Overwrite Value_/1 -> ISignal Overwrite Value/1  "ISignal Overwrite Value"
  Const_sigRMSCurrent Overwrite Value/1 -> _ISignal Overwrite Value_/1  "sigRMSCurrent Overwrite Value"

== system DriveSystemControl/Bus Configuration (1) - In/Manipulation/Virya Controller CAN File 08082024/WIP/CANChannel/PDUs/TCU01/sigSpeed/Feature Switch ==
  Const_sigSpeed Countdown Start Value : Constant  Value=0  OutDataTypeStr=uint32
  Const_sigSpeed Feature Switch : Constant  Value=0  OutDataTypeStr=uint32
  _Feature Switch_ : BusCreator  Inputs=2
  Feature Switch : Outport
  wires:
  _Feature Switch_/1 -> Feature Switch/1  "Feature Switch"
  Const_sigSpeed Countdown Start Value/1 -> _Feature Switch_/1  "sigSpeed Countdown Start Value"
  Const_sigSpeed Feature Switch/1 -> _Feature Switch_/2  "sigSpeed Feature Switch"

== system DriveSystemControl/Bus Configuration (1) - In/Manipulation/Virya Controller CAN File 08082024/WIP/CANChannel/PDUs/TCU01/sigSpeed/ISignal Overwrite Value ==
  Const_sigSpeed Overwrite Value : Constant  Value=0  OutDataTypeStr=uint8
  _ISignal Overwrite Value_ : BusCreator  Inputs=1
  ISignal Overwrite Value : Outport
  wires:
  _ISignal Overwrite Value_/1 -> ISignal Overwrite Value/1  "ISignal Overwrite Value"
  Const_sigSpeed Overwrite Value/1 -> _ISignal Overwrite Value_/1  "sigSpeed Overwrite Value"

== system DriveSystemControl/Bus Configuration (1) - In/Manipulation/Virya Controller CAN File 08082024/WIP/CANChannel/PDUs/TCU01/sigThrottle/Feature Switch ==
  Const_sigThrottle Countdown Start Value : Constant  Value=0  OutDataTypeStr=uint32
  Const_sigThrottle Feature Switch : Constant  Value=0  OutDataTypeStr=uint32
  _Feature Switch_ : BusCreator  Inputs=2
  Feature Switch : Outport
  wires:
  _Feature Switch_/1 -> Feature Switch/1  "Feature Switch"
  Const_sigThrottle Countdown Start Value/1 -> _Feature Switch_/1  "sigThrottle Countdown Start Value"
  Const_sigThrottle Feature Switch/1 -> _Feature Switch_/2  "sigThrottle Feature Switch"

== system DriveSystemControl/Bus Configuration (1) - In/Manipulation/Virya Controller CAN File 08082024/WIP/CANChannel/PDUs/TCU01/sigThrottle/ISignal Overwrite Value ==
  Const_sigThrottle Overwrite Value : Constant  Value=0  OutDataTypeStr=uint8
  _ISignal Overwrite Value_ : BusCreator  Inputs=1
  ISignal Overwrite Value : Outport
  wires:
  _ISignal Overwrite Value_/1 -> ISignal Overwrite Value/1  "ISignal Overwrite Value"
  Const_sigThrottle Overwrite Value/1 -> _ISignal Overwrite Value_/1  "sigThrottle Overwrite Value"

== system DriveSystemControl/Bus Configuration (1) - In/Manipulation/Virya Controller CAN File 08082024/WIP/CANChannel/PDUs/TCU02/sigCapacitorVoltage/Feature Switch ==
  Const_sigCapacitorVoltage Countdown Start Value : Constant  Value=0  OutDataTypeStr=uint32
  Const_sigCapacitorVoltage Feature Switch : Constant  Value=0  OutDataTypeStr=uint32
  _Feature Switch_ : BusCreator  Inputs=2
  Feature Switch : Outport
  wires:
  _Feature Switch_/1 -> Feature Switch/1  "Feature Switch"
  Const_sigCapacitorVoltage Countdown Start Value/1 -> _Feature Switch_/1  "sigCapacitorVoltage Countdown Start Value"
  Const_sigCapacitorVoltage Feature Switch/1 -> _Feature Switch_/2  "sigCapacitorVoltage Feature Switch"

== system DriveSystemControl/Bus Configuration (1) - In/Manipulation/Virya Controller CAN File 08082024/WIP/CANChannel/PDUs/TCU02/sigCapacitorVoltage/ISignal Overwrite Value ==
  Const_sigCapacitorVoltage Overwrite Value : Constant  Value=0  OutDataTypeStr=double
  _ISignal Overwrite Value_ : BusCreator  Inputs=1
  ISignal Overwrite Value : Outport
  wires:
  _ISignal Overwrite Value_/1 -> ISignal Overwrite Value/1  "ISignal Overwrite Value"
  Const_sigCapacitorVoltage Overwrite Value/1 -> _ISignal Overwrite Value_/1  "sigCapacitorVoltage Overwrite Value"

== system DriveSystemControl/Bus Configuration (1) - In/Manipulation/Virya Controller CAN File 08082024/WIP/CANChannel/PDUs/TCU02/sigMotorRPM/Feature Switch ==
  Const_sigMotorRPM Countdown Start Value : Constant  Value=0  OutDataTypeStr=uint32
  Const_sigMotorRPM Feature Switch : Constant  Value=0  OutDataTypeStr=uint32
  _Feature Switch_ : BusCreator  Inputs=2
  Feature Switch : Outport
  wires:
  _Feature Switch_/1 -> Feature Switch/1  "Feature Switch"
  Const_sigMotorRPM Countdown Start Value/1 -> _Feature Switch_/1  "sigMotorRPM Countdown Start Value"
  Const_sigMotorRPM Feature Switch/1 -> _Feature Switch_/2  "sigMotorRPM Feature Switch"

== system DriveSystemControl/Bus Configuration (1) - In/Manipulation/Virya Controller CAN File 08082024/WIP/CANChannel/PDUs/TCU02/sigMotorRPM/ISignal Overwrite Value ==
  Const_sigMotorRPM Overwrite Value : Constant  Value=0  OutDataTypeStr=int16
  _ISignal Overwrite Value_ : BusCreator  Inputs=1
  ISignal Overwrite Value : Outport
  wires:
  _ISignal Overwrite Value_/1 -> ISignal Overwrite Value/1  "ISignal Overwrite Value"
  Const_sigMotorRPM Overwrite Value/1 -> _ISignal Overwrite Value_/1  "sigMotorRPM Overwrite Value"

== system DriveSystemControl/Bus Configuration (1) - In/Manipulation/Virya Controller CAN File 08082024/WIP/CANChannel/PDUs/TCU02/sigOdometer/Feature Switch ==
  Const_sigOdometer Countdown Start Value : Constant  Value=0  OutDataTypeStr=uint32
  Const_sigOdometer Feature Switch : Constant  Value=0  OutDataTypeStr=uint32
  _Feature Switch_ : BusCreator  Inputs=2
  Feature Switch : Outport
  wires:
  _Feature Switch_/1 -> Feature Switch/1  "Feature Switch"
  Const_sigOdometer Countdown Start Value/1 -> _Feature Switch_/1  "sigOdometer Countdown Start Value"
  Const_sigOdometer Feature Switch/1 -> _Feature Switch_/2  "sigOdometer Feature Switch"

== system DriveSystemControl/Bus Configuration (1) - In/Manipulation/Virya Controller CAN File 08082024/WIP/CANChannel/PDUs/TCU02/sigOdometer/ISignal Overwrite Value ==
  Const_sigOdometer Overwrite Value : Constant  Value=0  OutDataTypeStr=double
  _ISignal Overwrite Value_ : BusCreator  Inputs=1
  ISignal Overwrite Value : Outport
  wires:
  _ISignal Overwrite Value_/1 -> ISignal Overwrite Value/1  "ISignal Overwrite Value"
  Const_sigOdometer Overwrite Value/1 -> _ISignal Overwrite Value_/1  "sigOdometer Overwrite Value"

== system DriveSystemControl/Bus Configuration (1) - In/Manipulation/Virya Controller CAN File 08082024/WIP/CANChannel/PDUs/TCU03/Controller_CompleteFaults/Feature Switch ==
  Const_Controller_CompleteFaults Countdown Start Value : Constant  Value=0  OutDataTypeStr=uint32
  Const_Controller_CompleteFaults Feature Switch : Constant  Value=0  OutDataTypeStr=uint32
  _Feature Switch_ : BusCreator  Inputs=2
  Feature Switch : Outport
  wires:
  _Feature Switch_/1 -> Feature Switch/1  "Feature Switch"
  Const_Controller_CompleteFaults Countdown Start Value/1 -> _Feature Switch_/1  "Controller_CompleteFaults Countdown Start Value"
  Const_Controller_CompleteFaults Feature Switch/1 -> _Feature Switch_/2  "Controller_CompleteFaults Feature Switch"

== system DriveSystemControl/Bus Configuration (1) - In/Manipulation/Virya Controller CAN File 08082024/WIP/CANChannel/PDUs/TCU03/Controller_CompleteFaults/ISignal Overwrite Value ==
  Const_Controller_CompleteFaults Overwrite Value : Constant  Value=0  OutDataTypeStr=uint8
  _ISignal Overwrite Value_ : BusCreator  Inputs=1
  ISignal Overwrite Value : Outport
  wires:
  _ISignal Overwrite Value_/1 -> ISignal Overwrite Value/1  "ISignal Overwrite Value"
  Const_Controller_CompleteFaults Overwrite Value/1 -> _ISignal Overwrite Value_/1  "Controller_CompleteFaults Overwrite Value"

== system DriveSystemControl/Bus Configuration (1) - In/Manipulation/Virya Controller CAN File 08082024/WIP/CANChannel/PDUs/TCU03/sig5VSupplyFailure/Feature Switch ==
  Const_sig5VSupplyFailure Countdown Start Value : Constant  Value=0  OutDataTypeStr=uint32
  Const_sig5VSupplyFailure Feature Switch : Constant  Value=0  OutDataTypeStr=uint32
  _Feature Switch_ : BusCreator  Inputs=2
  Feature Switch : Outport
  wires:
  _Feature Switch_/1 -> Feature Switch/1  "Feature Switch"
  Const_sig5VSupplyFailure Countdown Start Value/1 -> _Feature Switch_/1  "sig5VSupplyFailure Countdown Start Value"
  Const_sig5VSupplyFailure Feature Switch/1 -> _Feature Switch_/2  "sig5VSupplyFailure Feature Switch"

== system DriveSystemControl/Bus Configuration (1) - In/Manipulation/Virya Controller CAN File 08082024/WIP/CANChannel/PDUs/TCU03/sig5VSupplyFailure/ISignal Overwrite Value ==
  Const_sig5VSupplyFailure Overwrite Value : Constant  Value=0  OutDataTypeStr=uint8
  _ISignal Overwrite Value_ : BusCreator  Inputs=1
  ISignal Overwrite Value : Outport
  wires:
  _ISignal Overwrite Value_/1 -> ISignal Overwrite Value/1  "ISignal Overwrite Value"
  Const_sig5VSupplyFailure Overwrite Value/1 -> _ISignal Overwrite Value_/1  "sig5VSupplyFailure Overwrite Value"
